simulink model "mdl2"  (Simulink 8.1)
settings: Solver=FixedStepDiscrete  SolverMode=SingleTasking  StartTime=TIME(1)  StopTime=TIME(end)  FixedStep=SIMSTEP  RelTol=1e-3
model workspace (MAT data in the model file):
  autoc_mdd_data01 : struct (value not decoded)
PreLoadFcn:
  | run('C:\Users\yoshi12\Documents\lab_yoshi\matlab\20150408_BenchMarkModel\auto_set.m');
  | load('scr_simdata_all.mat');
  | load('scr_simdata.mat');
undefined symbols (not defined in the file): Parameter144, Parameter25, Parameter29, Parameter33, Parameter35, Parameter38, Parameter41, Parameter43, Parameter45, Parameter48, Parameter51, Parameter52, Parameter53, SIMSTEP
libraries: lib_all x9
settings Model: autoc_cdm_savetype=ModelWorkspace  autoc_cdm_name=autoc_mdd_data01  autoc_current_model=mdl2  autoc_dsminitmode=spec  Creator=905900  LastModifiedBy=yoshi12
settings OptimizationCC: BooleanDataType=off  InlineParams=on  InlineInvariantSignals=on  UseTempVars=on  InitFltsAndDblsToZero=on  OptimizeModelRefInitCode=on  LifeSpan=1
settings DebuggingCC: SignalInfNanChecking=warning  SaveWithParameterizedLinksMsg=none  CheckExecutionContextPreStartOutputMsg=on  CheckExecutionContextRuntimeOutputMsg=on  TimeAdjustmentMsg=warning  SolverPrmCheckMsg=none  InheritedTsInSrcMsg=none  MultiTaskDSMMsg=warning  MultiTaskCondExecSysMsg=none  TasksWithSamePriorityMsg=none  UnconnectedInputMsg=error  UnconnectedOutputMsg=error  UnconnectedLineMsg=error  UniqueDataStoreMsg=error  BusObjectLabelMismatch=error  RootOutportRequireBusObject=error  ModelReferenceIOMsg=warning  ModelReferenceVersionMismatchMessage=warning  ModelReferenceIOMismatchMessage=warning  StrictBusMsg=Warning
settings HardwareCC: ProdIntDivRoundTo=Floor  ProdEndianess=LittleEndian  ProdHWDeviceType=Specified  TargetHWDeviceType=32-bit Generic  ProdEqTarget=off
settings ModelReferenceCC: ModelReferenceNumInstancesAllowed=Single
settings SFSimCC: SimParseCustomCode=off
settings RTWCC: SystemTargetFile=ert.tlc  GenCodeOnly=on  TemplateMakefile=ert_default_tmf  Description=Real-Time Workshop Embedded Coder (no auto configuration)  RTWVerbose=off  ProcessScript=ert_make_rtw_hook
settings CodeAppCC: ForceParamTrailComments=on  IgnoreCustomStorageClasses=off  CustomSymbolStrType=$N$R$M  InternalIdentifier=Classic
settings ERTTargetCC: TargetFcnLib=ansi_tfl_tmw.mat  CodeReplacementLibrary=ANSI_C  MultiwordLength=2048  GenerateSampleERTMain=on  InlinedParameterPlacement=NonHierarchical  ERTCustomFileTemplate=example_file_process.tlc  ConvertIfToSwitch=off  SuppressUnreachableDefaultCases=off

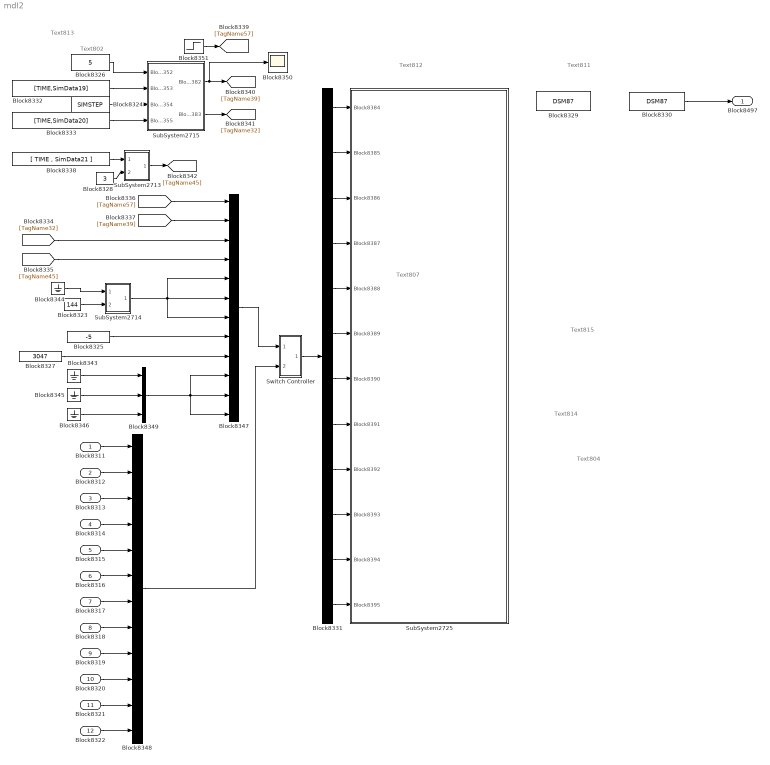
== system mdl2 ==
  note: Text815
  note: Text814
  note: Text813
  note: Text812
  note: Text811
  note: Text807
  note: Text804
  note: Text802
  Block8311 : Inport  SampleTime=SIMSTEP
  Block8312 : Inport  Port=2  SampleTime=SIMSTEP
  Block8313 : Inport  Port=3  PortDimensions=1
  Block8314 : Inport  Port=4  PortDimensions=3
  Block8315 : Inport  Port=5  PortDimensions=144
  Block8316 : Inport  Port=6  PortDimensions=144
  Block8317 : Inport  Port=7  PortDimensions=144
  Block8318 : Inport  Port=8  PortDimensions=1
  Block8319 : Inport  Port=9  PortDimensions=1
  Block8320 : Inport  Port=10  PortDimensions=3
  Block8321 : Inport  Port=11  PortDimensions=3
  Block8322 : Inport  Port=12  PortDimensions=3
  Block8323 : Constant  Value=144  OutDataTypeStr=double  SampleTime=-1
  Block8324 : Constant  Value=SIMSTEP  OutDataTypeStr=double  SampleTime=-1
  Block8325 : Constant  Value=-5  OutDataTypeStr=double  SampleTime=SIMSTEP
  Block8326 : Constant  Value=5  OutDataTypeStr=double  SampleTime=-1
  Block8327 : Constant  Value=3047  OutDataTypeStr=double  SampleTime=-1
  Block8328 : Constant  Value=3  OutDataTypeStr=double  SampleTime=-1
  Block8329 : DataStoreMemory  DataStoreName=DSM87  InitialValue=[0 0 0]  OutDataTypeStr=double
  Block8330 : DataStoreRead  DataStoreName=DSM87
  Block8331 : Demux  Outputs=12
  Block8332 : FromWorkspace  VariableName=[TIME,SimData19]  SampleTime=SIMSTEP
  Block8333 : FromWorkspace  VariableName=[TIME,SimData20]  SampleTime=SIMSTEP  Interpolate=off  OutputAfterFinalValue=Holding final value
  Block8338 : FromWorkspace  VariableName=[ TIME , SimData21 ]  SampleTime=SIMSTEP  Interpolate=off  OutputAfterFinalValue=Holding final value
  Block{8343..8346} (4 alike) : Ground
  Block8347 : Mux  Inputs=12
  Block8348 : Mux  Inputs=12
  Block8349 : Mux  Inputs=3
  Block8350 : Scope
      settings: YMin=0  YMax=1
  Block8351 : Step  Time=SIMSTEP  SampleTime=SIMSTEP
  SubSystem2713 : Subsystem
  SubSystem2714 : Subsystem
  SubSystem2715 : Subsystem
  SubSystem2725 : Subsystem
  Switch Controller : Subsystem  mask(Switch Controller){}
      mask init:
      | if strcmpi(get_param(bdroot(gcbh), 'ModelReferenceTargetType'), 'SIM')
      |     % During simulation, data source for unit model is coming from parent model
      |     mode = false;
      | else
      |     mode = true;
      | end
      | switch_mode = mode;
      settings: OpenFcn="msgbox(['1. モデル単体でのシミュレーション時，In端子を出力します．' 10 10 '2. Model Reference経由で起動時，MR_In端子を出力します．' 10 10 10 '  ■注意：モデルの表紙ページでのみ使用してください．'], 'Switch Controller');"
  Block8497 : Outport
  wires:
  Block8330/1 -> Block8497/1
  Block8331/1 -> SubSystem2725/1(Block8384)
  Block8331/2 -> SubSystem2725/2(Block8385)
  Block8331/3 -> SubSystem2725/3(Block8386)
  Block8331/4 -> SubSystem2725/4(Block8387)
  Block8331/5 -> SubSystem2725/5(Block8388)
  Block8331/6 -> SubSystem2725/6(Block8389)
  Block8331/7 -> SubSystem2725/7(Block8390)
  Block8331/8 -> SubSystem2725/8(Block8391)
  Block8331/9 -> SubSystem2725/9(Block8392)
  Block8331/10 -> SubSystem2725/10(Block8393)
  Block8331/11 -> SubSystem2725/11(Block8394)
  Block8331/12 -> SubSystem2725/12(Block8395)
  Switch Controller/1(Out) -> Block8331/1
  Block8311/1 -> Block8348/1
  Block8312/1 -> Block8348/2
  Block8313/1 -> Block8348/3
  Block8314/1 -> Block8348/4
  Block8315/1 -> Block8348/5
  Block8316/1 -> Block8348/6
  Block8317/1 -> Block8348/7
  Block8318/1 -> Block8348/8
  Block8319/1 -> Block8348/9
  Block8320/1 -> Block8348/10
  Block8321/1 -> Block8348/11
  Block8322/1 -> Block8348/12
  Block8347/1 -> Switch Controller/1(In)
  Block8348/1 -> Switch Controller/2(MR_In)
  [TagName45] -> Block8347/4
  Block8327/1 -> Block8347/9
  [TagName32] -> Block8347/3
  Block8325/1 -> Block8347/8
  Block8343/1 -> Block8349/1
  Block8345/1 -> Block8349/2
  Block8346/1 -> Block8349/3
  Block8349/1 -> Block8347/11, Block8347/10, Block8347/12
  Block8338/1 -> SubSystem2713/1(Scalar)
  SubSystem2713/1(Vector) -> [TagName45]
  Block8328/1 -> SubSystem2713/2(Width)
  [TagName57] -> Block8347/1
  [TagName39] -> Block8347/2
  SubSystem2714/1(Vector) -> Block8347/6, Block8347/7, Block8347/5
  Block8344/1 -> SubSystem2714/1(Scalar)
  Block8323/1 -> SubSystem2714/2(Width)
  Block8351/1 -> [TagName57]
  Block8332/1 -> SubSystem2715/2(Block8353)
  Block8324/1 -> SubSystem2715/3(Block8354)
  SubSystem2715/2(Block8383) -> [TagName32]
  Block8333/1 -> SubSystem2715/4(Block8355)
  Block8326/1 -> SubSystem2715/1(Block8352)
  SubSystem2715/1(Block8382) -> [TagName39], Block8350/1

== system mdl2/SubSystem2713 ==
  note: ***編集禁止***
  Scalar : Inport
  Width : Inport  Port=2
  Mux : Mux  Inputs=3
  Terminator : Terminator
  Vector : Outport
  wires:
  Width/1 -> Terminator/1
  Mux/1 -> Vector/1
  Scalar/1 -> Mux/1, Mux/2, Mux/3

== system mdl2/SubSystem2714 ==
  note: ***編集禁止***
  Scalar : Inport
  Width : Inport  Port=2
  Mux : Mux  Inputs=144
  Terminator : Terminator
  Vector : Outport
  wires:
  Mux/1 -> Vector/1
  Width/1 -> Terminator/1
  Scalar/1 -> Mux/1, Mux/2, Mux/3, Mux/4, Mux/5, Mux/6, Mux/7, Mux/8, Mux/9, Mux/10, Mux/11, Mux/12, Mux/13, Mux/14, Mux/15, Mux/16, Mux/17, Mux/18, Mux/19, Mux/20, Mux/21, Mux/22, Mux/23, Mux/24, Mux/25, Mux/26, Mux/27, Mux/28, Mux/29, Mux/30, Mux/31, Mux/32, Mux/33, Mux/34, Mux/35, Mux/36, Mux/37, Mux/38, Mux/39, Mux/40, Mux/41, Mux/42, Mux/43, Mux/44, Mux/45, Mux/46, Mux/47, Mux/48, Mux/49, Mux/50, Mux/51, Mux/52, Mux/53, Mux/54, Mux/55, Mux/56, Mux/57, Mux/58, Mux/59, Mux/60, Mux/61, Mux/62, Mux/63, Mux/64, Mux/65, Mux/66, Mux/67, Mux/68, Mux/69, Mux/70, Mux/71, Mux/72, Mux/73, Mux/74, Mux/75, Mux/76, Mux/77, Mux/78, Mux/79, Mux/80, Mux/81, Mux/82, Mux/83, Mux/84, Mux/85, Mux/86, Mux/87, Mux/88, Mux/89, Mux/90, Mux/91, Mux/92, Mux/93, Mux/94, Mux/95, Mux/96, Mux/97, Mux/98, Mux/99, Mux/100, Mux/101, Mux/102, Mux/103, Mux/104, Mux/105, Mux/106, Mux/107, Mux/108, Mux/109, Mux/110, Mux/111, Mux/112, Mux/113, Mux/114, Mux/115, Mux/116, Mux/117, Mux/118, Mux/119, Mux/120, Mux/121, Mux/122, Mux/123, Mux/124, Mux/125, Mux/126, Mux/127, Mux/128, Mux/129, Mux/130, Mux/131, Mux/132, Mux/133, Mux/134, Mux/135, Mux/136, Mux/137, Mux/138, Mux/139, Mux/140, Mux/141, Mux/142, Mux/143, Mux/144

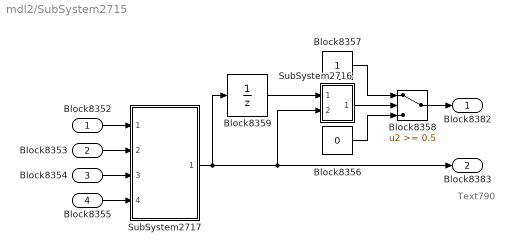
== system mdl2/SubSystem2715 ==
  note: Text790
  Block8352 : Inport
  Block8353 : Inport  Port=2
  Block8354 : Inport  Port=3
  Block8355 : Inport  Port=4
  Block8356 : Constant  Value=0  OutDataTypeStr=double  SampleTime=-1
  Block8357 : Constant  OutDataTypeStr=double  SampleTime=-1
  Block8358 : Switch  Threshold=0.5  RndMeth=Zero  SaturateOnIntegerOverflow=on  InputSameDT=on
  Block8359 : UnitDelay  SampleTime=-1
  SubSystem2716 : Subsystem
  SubSystem2717 : Subsystem
  Block8382 : Outport
  Block8383 : Outport  Port=2
  wires:
  SubSystem2717/1(Block8381) -> Block8359/1, Block8383/1, SubSystem2716/2(In2)
  Block8359/1 -> SubSystem2716/1(In1)
  SubSystem2716/1(Out1) -> Block8358/2
  Block8357/1 -> Block8358/1
  Block8356/1 -> Block8358/3
  Block8358/1 -> Block8382/1
  Block8353/1 -> SubSystem2717/2(Block8361)
  Block8354/1 -> SubSystem2717/3(Block8362)
  Block8355/1 -> SubSystem2717/4(Block8363)
  Block8352/1 -> SubSystem2717/1(Block8360)

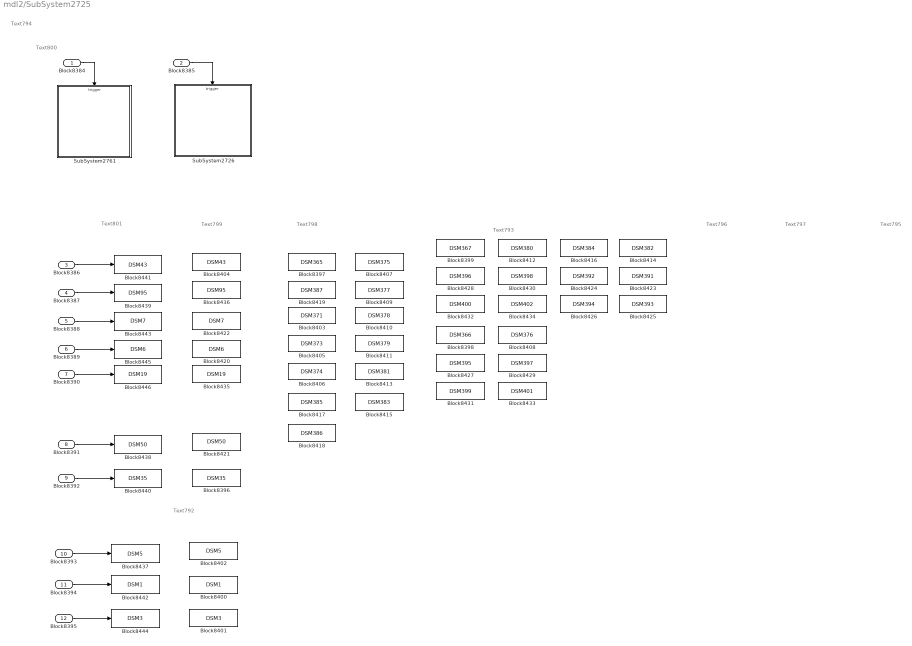
== system mdl2/SubSystem2725 ==
  note: Text801
  note: Text800
  note: Text799
  note: Text798
  note: Text797
  note: Text796
  note: Text795
  note: Text794
  note: Text793
  note: Text792
  Block8384 : Inport
  Block8385 : Inport  Port=2
  Block8386 : Inport  Port=3
  Block8387 : Inport  Port=4
  Block8388 : Inport  Port=5
  Block8389 : Inport  Port=6
  Block8390 : Inport  Port=7
  Block8391 : Inport  Port=8
  Block8392 : Inport  Port=9
  Block8393 : Inport  Port=10
  Block8394 : Inport  Port=11
  Block8395 : Inport  Port=12
  Block8396 : DataStoreMemory  DataStoreName=DSM35  OutDataTypeStr=double
  Block8397 : DataStoreMemory  DataStoreName=DSM365  OutDataTypeStr=double
  Block8398 : DataStoreMemory  DataStoreName=DSM366  InitialValue=[0 0 0 0 0 0 0 0 0 0 0 0 0 0 0 0 0 0 0 0 0 0 0 0 0 0 0 0 0 0 0 0 0 0 0 0 0 0 0 0 0 0 0 0 0 0 0 0 0 0 0 0 0 0 0 0 0 0 0 0 0 0 0 0 0 0 0 0 0 0 0 0 0 0 0 0 0 0 0 0 0 0 0 0 0 0 0 0 0 0 0 0 0 0 0 0 0 0 0 0 0 0 0 0 0 0 0 0 0 0 0 0 0 0 0 0 0 0 0 0 0 0 0 0 0 0 0 0]  OutDataTypeStr=double
  Block8399 : DataStoreMemory  DataStoreName=DSM367  InitialValue=[0 0 0 0 0 0 0 0 0 0 0 0 0 0 0 0 0 0 0 0 0 0 0 0 0 0 0 0 0 0 0 0 0 0 0 0 0 0 0 0 0 0 0 0 0 0 0 0 0 0 0 0 0 0 0 0 0 0 0 0 0 0 0 0 0 0 0 0 0 0 0 0 0 0 0 0 0 0 0 0 0 0 0 0 0 0 0 0 0 0 0 0 0 0 0 0 0 0 0 0 0 0 0 0 0 0 0 0 0 0 0 0 0 0 0 0 0 0 0 0 0 0 0 0 0 0 0 0]  OutDataTypeStr=double
  Block8400 : DataStoreMemory  DataStoreName=DSM1  InitialValue=[0 0 0]  OutDataTypeStr=double
  Block8401 : DataStoreMemory  DataStoreName=DSM3  InitialValue=[0 0 0]  OutDataTypeStr=double
  Block8402 : DataStoreMemory  DataStoreName=DSM5  InitialValue=[0 0 0]  OutDataTypeStr=double
  Block8403 : DataStoreMemory  DataStoreName=DSM371  InitialValue=[0 0 0]  OutDataTypeStr=double
  Block8404 : DataStoreMemory  DataStoreName=DSM43  OutDataTypeStr=double
  Block8405 : DataStoreMemory  DataStoreName=DSM373  InitialValue=[0 0 0]  OutDataTypeStr=double
  Block8406 : DataStoreMemory  DataStoreName=DSM374  InitialValue=[0 0 0]  OutDataTypeStr=double
  Block8407 : DataStoreMemory  DataStoreName=DSM375  InitialValue=[0 0 0]  OutDataTypeStr=double
  Block8408 : DataStoreMemory  DataStoreName=DSM376  InitialValue=[0 0 0 0 0 0 0 0 0 0 0 0 0 0 0 0]  OutDataTypeStr=double
  Block8409 : DataStoreMemory  DataStoreName=DSM377  InitialValue=[0 0 0]  OutDataTypeStr=double
  Block8410 : DataStoreMemory  DataStoreName=DSM378  InitialValue=[0 0 0]  OutDataTypeStr=double
  Block8411 : DataStoreMemory  DataStoreName=DSM379  InitialValue=[0 0 0]  OutDataTypeStr=double
  Block8412 : DataStoreMemory  DataStoreName=DSM380  InitialValue=[0 0 0 0 0 0 0 0 0 0 0 0 0 0 0 0]  OutDataTypeStr=double
  Block8413 : DataStoreMemory  DataStoreName=DSM381  InitialValue=[0 0 0]  OutDataTypeStr=double
  Block8414 : DataStoreMemory  DataStoreName=DSM382  InitialValue=[0 0 0 0 0 0 0 0 0 0 0 0 0 0 0 0 0 0 0 0 0 0 0 0 0 0 0 0 0 0 0 0 0 0 0 0 0 0 0 0 0 0 0 0 0 0 0 0 0 0 0 0 0 0 0 0 0 0 0 0 0 0 0 0 0 0 0 0 0 0 0 0 0 0 0 0 0 0 0 0 0 0 0 0 0 0 0 0 0 0 0 0 0 0 0 0 0 0 0 0 0 0 0 0 0 0 0 0 0 0 0 0 0 0 0 0 0 0 0 0 0 0 0 0 0 0 0 0]  OutDataTypeStr=double
  Block8415 : DataStoreMemory  DataStoreName=DSM383  InitialValue=[0 0 0]  OutDataTypeStr=double
  Block8416 : DataStoreMemory  DataStoreName=DSM384  InitialValue=[0 0 0 0 0 0 0 0 0 0 0 0 0 0 0 0 0 0 0 0 0 0 0 0 0 0 0 0 0 0 0 0 0 0 0 0 0 0 0 0 0 0 0 0 0 0 0 0 0 0 0 0 0 0 0 0 0 0 0 0 0 0 0 0 0 0 0 0 0 0 0 0 0 0 0 0 0 0 0 0 0 0 0 0 0 0 0 0 0 0 0 0 0 0 0 0 0 0 0 0 0 0 0 0 0 0 0 0 0 0 0 0 0 0 0 0 0 0 0 0 0 0 0 0 0 0 0 0]  OutDataTypeStr=double
  Block8417 : DataStoreMemory  DataStoreName=DSM385  InitialValue=[0 0 0]  OutDataTypeStr=double
  Block8418 : DataStoreMemory  DataStoreName=DSM386  InitialValue=[0 0 0]  OutDataTypeStr=double
  Block8419 : DataStoreMemory  DataStoreName=DSM387  InitialValue=[0 0 0]  OutDataTypeStr=double
  Block8420 : DataStoreMemory  DataStoreName=DSM6  InitialValue=[0 0 0 0 0 0 0 0 0 0 0 0 0 0 0 0 0 0 0 0 0 0 0 0 0 0 0 0 0 0 0 0 0 0 0 0 0 0 0 0 0 0 0 0 0 0 0 0 0 0 0 0 0 0 0 0 0 0 0 0 0 0 0 0 0 0 0 0 0 0 0 0 0 0 0 0 0 0 0 0 0 0 0 0 0 0 0 0 0 0 0 0 0 0 0 0 0 0 0 0 0 0 0 0 0 0 0 0 0 0 0 0 0 0 0 0 0 0 0 0 0 0 0 0 0 0 0 0 0 0 0 0 0 0 0 0 0 0 0 0 0 0 0 0]  OutDataTypeStr=double
  Block8421 : DataStoreMemory  DataStoreName=DSM50  OutDataTypeStr=double
  Block8422 : DataStoreMemory  DataStoreName=DSM7  InitialValue=[0 0 0 0 0 0 0 0 0 0 0 0 0 0 0 0 0 0 0 0 0 0 0 0 0 0 0 0 0 0 0 0 0 0 0 0 0 0 0 0 0 0 0 0 0 0 0 0 0 0 0 0 0 0 0 0 0 0 0 0 0 0 0 0 0 0 0 0 0 0 0 0 0 0 0 0 0 0 0 0 0 0 0 0 0 0 0 0 0 0 0 0 0 0 0 0 0 0 0 0 0 0 0 0 0 0 0 0 0 0 0 0 0 0 0 0 0 0 0 0 0 0 0 0 0 0 0 0 0 0 0 0 0 0 0 0 0 0 0 0 0 0 0 0]  OutDataTypeStr=double
  Block8423 : DataStoreMemory  DataStoreName=DSM391  InitialValue=[0 0 0 0 0 0 0 0 0 0 0 0 0 0 0 0 0 0 0 0 0 0 0 0 0 0 0 0 0 0 0 0 0 0 0 0 0 0 0 0 0 0 0 0 0 0 0 0 0 0 0 0 0 0 0 0 0 0 0 0 0 0 0 0 0 0 0 0 0 0 0 0 0 0 0 0 0 0 0 0 0 0 0 0 0 0 0 0 0 0 0 0 0 0 0 0 0 0 0 0 0 0 0 0 0 0 0 0 0 0 0 0 0 0 0 0 0 0 0 0 0 0 0 0 0 0 0 0]  OutDataTypeStr=double
  Block8424 : DataStoreMemory  DataStoreName=DSM392  InitialValue=[0 0 0 0 0 0 0 0 0 0 0 0 0 0 0 0 0 0 0 0 0 0 0 0 0 0 0 0 0 0 0 0 0 0 0 0 0 0 0 0 0 0 0 0 0 0 0 0 0 0 0 0 0 0 0 0 0 0 0 0 0 0 0 0 0 0 0 0 0 0 0 0 0 0 0 0 0 0 0 0 0 0 0 0 0 0 0 0 0 0 0 0 0 0 0 0 0 0 0 0 0 0 0 0 0 0 0 0 0 0 0 0 0 0 0 0 0 0 0 0 0 0 0 0 0 0 0 0]  OutDataTypeStr=double
  Block8425 : DataStoreMemory  DataStoreName=DSM393  InitialValue=[0 0 0 0 0 0 0 0 0 0 0 0 0 0 0 0 0 0 0 0 0 0 0 0 0 0 0 0 0 0 0 0 0 0 0 0 0 0 0 0 0 0 0 0 0 0 0 0 0 0 0 0 0 0 0 0 0 0 0 0 0 0 0 0 0 0 0 0 0 0 0 0 0 0 0 0 0 0 0 0 0 0 0 0 0 0 0 0 0 0 0 0 0 0 0 0 0 0 0 0 0 0 0 0 0 0 0 0 0 0 0 0 0 0 0 0 0 0 0 0 0 0 0 0 0 0 0 0]  OutDataTypeStr=double
  Block8426 : DataStoreMemory  DataStoreName=DSM394  InitialValue=[0 0 0 0 0 0 0 0 0 0 0 0 0 0 0 0 0 0 0 0 0 0 0 0 0 0 0 0 0 0 0 0 0 0 0 0 0 0 0 0 0 0 0 0 0 0 0 0 0 0 0 0 0 0 0 0 0 0 0 0 0 0 0 0 0 0 0 0 0 0 0 0 0 0 0 0 0 0 0 0 0 0 0 0 0 0 0 0 0 0 0 0 0 0 0 0 0 0 0 0 0 0 0 0 0 0 0 0 0 0 0 0 0 0 0 0 0 0 0 0 0 0 0 0 0 0 0 0]  OutDataTypeStr=double
  Block8427 : DataStoreMemory  DataStoreName=DSM395  InitialValue=[0 0 0 0 0 0 0 0 0 0 0 0 0 0 0 0 0 0 0 0 0 0 0 0 0 0 0 0 0 0 0 0 0 0 0 0 0 0 0 0 0 0 0 0 0 0 0 0 0 0 0 0 0 0 0 0 0 0 0 0 0 0 0 0 0 0 0 0 0 0 0 0 0 0 0 0 0 0 0 0 0 0 0 0 0 0 0 0 0 0 0 0 0 0 0 0 0 0 0 0 0 0 0 0 0 0 0 0 0 0 0 0 0 0 0 0 0 0 0 0 0 0 0 0 0 0 0 0]  OutDataTypeStr=double
  Block8428 : DataStoreMemory  DataStoreName=DSM396  InitialValue=[0 0 0 0 0 0 0 0 0 0 0 0 0 0 0 0 0 0 0 0 0 0 0 0 0 0 0 0 0 0 0 0 0 0 0 0 0 0 0 0 0 0 0 0 0 0 0 0 0 0 0 0 0 0 0 0 0 0 0 0 0 0 0 0 0 0 0 0 0 0 0 0 0 0 0 0 0 0 0 0 0 0 0 0 0 0 0 0 0 0 0 0 0 0 0 0 0 0 0 0 0 0 0 0 0 0 0 0 0 0 0 0 0 0 0 0 0 0 0 0 0 0 0 0 0 0 0 0]  OutDataTypeStr=double
  Block8429 : DataStoreMemory  DataStoreName=DSM397  InitialValue=[0 0 0 0 0 0 0 0 0 0 0 0 0 0 0 0]  OutDataTypeStr=double
  Block8430 : DataStoreMemory  DataStoreName=DSM398  InitialValue=[0 0 0 0 0 0 0 0 0 0 0 0 0 0 0 0]  OutDataTypeStr=double
  Block8431 : DataStoreMemory  DataStoreName=DSM399  InitialValue=[0 0 0 0 0 0 0 0 0 0 0 0 0 0 0 0 0 0 0 0 0 0 0 0 0 0 0 0 0 0 0 0 0 0 0 0 0 0 0 0 0 0 0 0 0 0 0 0 0 0 0 0 0 0 0 0 0 0 0 0 0 0 0 0 0 0 0 0 0 0 0 0 0 0 0 0 0 0 0 0 0 0 0 0 0 0 0 0 0 0 0 0 0 0 0 0 0 0 0 0 0 0 0 0 0 0 0 0 0 0 0 0 0 0 0 0 0 0 0 0 0 0 0 0 0 0 0 0]  OutDataTypeStr=double
  Block8432 : DataStoreMemory  DataStoreName=DSM400  InitialValue=[0 0 0 0 0 0 0 0 0 0 0 0 0 0 0 0 0 0 0 0 0 0 0 0 0 0 0 0 0 0 0 0 0 0 0 0 0 0 0 0 0 0 0 0 0 0 0 0 0 0 0 0 0 0 0 0 0 0 0 0 0 0 0 0 0 0 0 0 0 0 0 0 0 0 0 0 0 0 0 0 0 0 0 0 0 0 0 0 0 0 0 0 0 0 0 0 0 0 0 0 0 0 0 0 0 0 0 0 0 0 0 0 0 0 0 0 0 0 0 0 0 0 0 0 0 0 0 0]  OutDataTypeStr=double
  Block8433 : DataStoreMemory  DataStoreName=DSM401  InitialValue=[0 0 0 0 0 0 0 0 0 0 0 0 0 0 0 0]  OutDataTypeStr=double
  Block8434 : DataStoreMemory  DataStoreName=DSM402  InitialValue=[0 0 0 0 0 0 0 0 0 0 0 0 0 0 0 0]  OutDataTypeStr=double
  Block8435 : DataStoreMemory  DataStoreName=DSM19  InitialValue=[0 0 0 0 0 0 0 0 0 0 0 0 0 0 0 0 0 0 0 0 0 0 0 0 0 0 0 0 0 0 0 0 0 0 0 0 0 0 0 0 0 0 0 0 0 0 0 0 0 0 0 0 0 0 0 0 0 0 0 0 0 0 0 0 0 0 0 0 0 0 0 0 0 0 0 0 0 0 0 0 0 0 0 0 0 0 0 0 0 0 0 0 0 0 0 0 0 0 0 0 0 0 0 0 0 0 0 0 0 0 0 0 0 0 0 0 0 0 0 0 0 0 0 0 0 0 0 0 0 0 0 0 0 0 0 0 0 0 0 0 0 0 0 0]  OutDataTypeStr=double
  Block8436 : DataStoreMemory  DataStoreName=DSM95  InitialValue=[0 0 0]  OutDataTypeStr=double
  Block8437 : DataStoreWrite  Priority=1  DataStoreName=DSM5
  Block8438 : DataStoreWrite  Priority=1  DataStoreName=DSM50
  Block8439 : DataStoreWrite  Priority=1  DataStoreName=DSM95
  Block8440 : DataStoreWrite  Priority=1  DataStoreName=DSM35
  Block8441 : DataStoreWrite  Priority=1  DataStoreName=DSM43
  Block8442 : DataStoreWrite  Priority=1  DataStoreName=DSM1
  Block8443 : DataStoreWrite  Priority=1  DataStoreName=DSM7
  Block8444 : DataStoreWrite  Priority=1  DataStoreName=DSM3
  Block8445 : DataStoreWrite  Priority=1  DataStoreName=DSM6
  Block8446 : DataStoreWrite  Priority=1  DataStoreName=DSM19
  SubSystem2726 : Subsystem  Priority=3  TreatAsAtomicUnit=on
      settings: AttributesFormatString=Attribute2234  RTWSystemCode=Nonreusable function  RTWFcnNameOpts=Use subsystem name
  SubSystem2761 : Subsystem  Priority=2  TreatAsAtomicUnit=on
      settings: AttributesFormatString=Attribute2268  RTWSystemCode=Nonreusable function  RTWFcnNameOpts=Use subsystem name
  wires:
  Block8385/1 -> SubSystem2726/Trigger
  Block8384/1 -> SubSystem2761/Trigger
  Block8387/1 -> Block8439/1
  Block8386/1 -> Block8441/1
  Block8391/1 -> Block8438/1
  Block8392/1 -> Block8440/1
  Block8388/1 -> Block8443/1
  Block8390/1 -> Block8446/1
  Block8389/1 -> Block8445/1
  Block8393/1 -> Block8437/1
  Block8394/1 -> Block8442/1
  Block8395/1 -> Block8444/1

== system mdl2/Switch Controller ==
  In : Inport  SampleTime=SIMSTEP
  MR_In : Inport  Port=2  SampleTime=SIMSTEP
  Numerical Unity : SignalConversion  ConversionOutput=Bus copy
  Sw1 : Switch  Threshold=0.5  SaturateOnIntegerOverflow=on  InputSameDT=on
  Switch Control : Constant  Value=switch_mode  OutDataTypeStr=boolean
  Out : Outport
  wires:
  In/1 -> Sw1/1
  Switch Control/1 -> Sw1/2
  Sw1/1 -> Numerical Unity/1
  MR_In/1 -> Sw1/3
  Numerical Unity/1 -> Out/1

== system mdl2/SubSystem2715/SubSystem2716 ==
  note: ***編集禁止***
  In1 : Inport
  In2 : Inport  Port=2
  RO1 : RelationalOperator  Operator=~=  InputSameDT=on
  single1 : DataTypeConversion  OutDataTypeStr=single  SaturateOnIntegerOverflow=on  RndMeth=Zero
  single2 : DataTypeConversion  OutDataTypeStr=single  SaturateOnIntegerOverflow=on  RndMeth=Zero
  Out1 : Outport
  wires:
  RO1/1 -> Out1/1
  In2/1 -> single2/1
  In1/1 -> single1/1
  single1/1 -> RO1/1
  single2/1 -> RO1/2

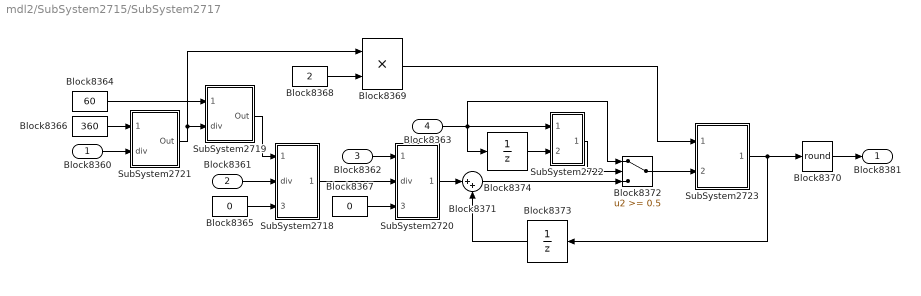
== system mdl2/SubSystem2715/SubSystem2717 ==
  Block8360 : Inport
  Block8361 : Inport  Port=2
  Block8362 : Inport  Port=3
  Block8363 : Inport  Port=4
  Block8364 : Constant  Value=60  OutDataTypeStr=double  SampleTime=-1
  Block8365 : Constant  Value=0  OutDataTypeStr=double  SampleTime=-1
  Block8366 : Constant  Value=360  OutDataTypeStr=double  SampleTime=-1
  Block8367 : Constant  Value=0  OutDataTypeStr=double  SampleTime=-1
  Block8368 : Constant  Value=2  OutDataTypeStr=double  SampleTime=-1
  Block8369 : Product  Inputs=**  SaturateOnIntegerOverflow=on  RndMeth=Zero  InputSameDT=on  OutDataTypeStr=Inherit: Same as first input
  Block8370 : Rounding  Operator=round
  Block8371 : Sum  Inputs=|++  OutDataTypeStr=double  RndMeth=Zero  SaturateOnIntegerOverflow=on  InputSameDT=on
  Block8372 : Switch  Threshold=0.5  RndMeth=Zero  SaturateOnIntegerOverflow=on  InputSameDT=on
  Block8373 : UnitDelay  SampleTime=-1
  Block8374 : UnitDelay  SampleTime=-1
  SubSystem2718 : Subsystem  TreatAsAtomicUnit=on  mask(***ATC.DIVISION***){bd_version=1.01.A, r0=チェック有り, r1=, r2=, r3=, r4=, r5=, r6=, r7=, r8=, r9=, c0=, c1=, c2=, c3=, c4=, c5=, c6=, c7=, c8=, c9=}
      mask prompts: bd_version "Version"
      mask help: これはAutoCからのブロックです．編集禁止．
      settings: OpenFcn=warndlg('変更禁止!');
      mask Help: web(ui_blockhelpmng(gcb));
  SubSystem2719 : Subsystem  TreatAsAtomicUnit=on  mask(***ATC.DIVISION***){bd_version=1.01.A, r0=チェック無し, r1=, r2=, r3=, r4=, r5=, r6=, r7=, r8=, r9=, c0=, c1=, c2=, c3=, c4=, c5=, c6=, c7=, c8=, c9=}
      mask prompts: bd_version "Version"
      mask help: これはAutoCからのブロックです．編集禁止．
      settings: OpenFcn=warndlg('変更禁止!');
      mask Help: web(ui_blockhelpmng(gcb));
  SubSystem2720 : Subsystem  TreatAsAtomicUnit=on  mask(***ATC.DIVISION***){bd_version=1.01.A, r0=チェック有り, r1=, r2=, r3=, r4=, r5=, r6=, r7=, r8=, r9=, c0=, c1=, c2=, c3=, c4=, c5=, c6=, c7=, c8=, c9=}
      mask prompts: bd_version "Version"
      mask help: これはAutoCからのブロックです．編集禁止．
      settings: OpenFcn=warndlg('変更禁止!');
      mask Help: web(ui_blockhelpmng(gcb));
  SubSystem2721 : Subsystem  TreatAsAtomicUnit=on  mask(***ATC.DIVISION***){bd_version=1.01.A, r0=チェック無し, r1=, r2=, r3=, r4=, r5=, r6=, r7=, r8=, r9=, c0=, c1=, c2=, c3=, c4=, c5=, c6=, c7=, c8=, c9=}
      mask prompts: bd_version "Version"
      mask help: これはAutoCからのブロックです．編集禁止．
      settings: OpenFcn=warndlg('変更禁止!');
      mask Help: web(ui_blockhelpmng(gcb));
  SubSystem2722 : Subsystem
  SubSystem2723 : Subsystem
      settings: RTWSystemCode=Inline
  Block8381 : Outport
  wires:
  Block8373/1 -> Block8371/2
  Block8371/1 -> Block8372/3
  Block8361/1 -> SubSystem2718/2(div)
  Block8365/1 -> SubSystem2718/3(init)
  Block8364/1 -> SubSystem2719/1(mult)
  SubSystem2719/1(Out) -> SubSystem2718/1(mult)
  SubSystem2720/1(Out) -> Block8371/1
  Block8362/1 -> SubSystem2720/1(mult)
  SubSystem2718/1(Out) -> SubSystem2720/2(div)
  Block8367/1 -> SubSystem2720/3(init)
  Block8370/1 -> Block8381/1
  SubSystem2722/1(Out1) -> Block8372/2
  Block8363/1 -> SubSystem2722/1(In1), Block8374/1, Block8372/1
  Block8374/1 -> SubSystem2722/2(In2)
  Block8372/1 -> SubSystem2723/2(Block8376)
  SubSystem2723/1(Block8380) -> Block8370/1, Block8373/1
  Block8366/1 -> SubSystem2721/1(mult)
  Block8360/1 -> SubSystem2721/2(div)
  Block8368/1 -> Block8369/2
  SubSystem2721/1(Out) -> SubSystem2719/2(div), Block8369/1
  Block8369/1 -> SubSystem2723/1(Block8375)

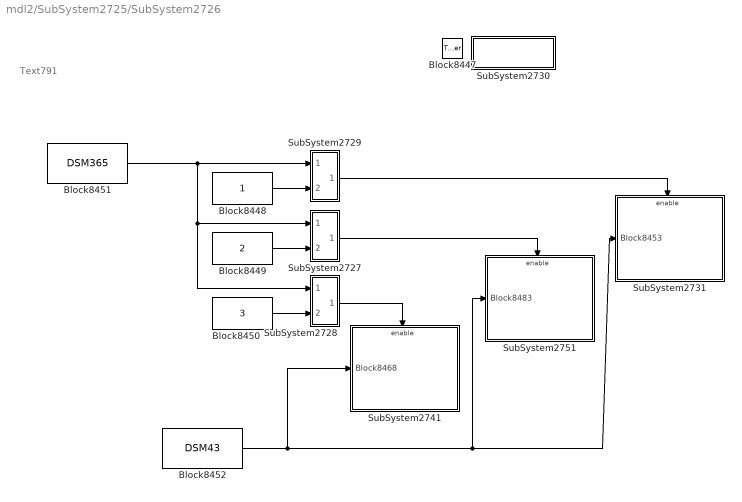
== system mdl2/SubSystem2725/SubSystem2726 ==
  note: Text791
  Block8447 : TriggerPort
  Block8448 : Constant  OutDataTypeStr=double  SampleTime=-1
  Block8449 : Constant  Value=2  OutDataTypeStr=double  SampleTime=-1
  Block8450 : Constant  Value=3  OutDataTypeStr=double  SampleTime=-1
  Block8451 : DataStoreRead  DataStoreName=DSM365
  Block8452 : DataStoreRead  DataStoreName=DSM43
  SubSystem2727 : Subsystem
  SubSystem2728 : Subsystem
  SubSystem2729 : Subsystem
  SubSystem2730 : Subsystem  mask(***ATC.TriggerFunction***){}
      mask help: これはAutoCからのブロックです．編集禁止．
      settings: AttributesFormatString=Attribute2238  OpenFcn=warndlg('変更禁止!');
      mask Display: disp('ATC.Trigger Function')
  SubSystem2731 : Subsystem  TreatAsAtomicUnit=on
  SubSystem2741 : Subsystem  TreatAsAtomicUnit=on
  SubSystem2751 : Subsystem  TreatAsAtomicUnit=on
  wires:
  Block8452/1 -> SubSystem2731/1(Block8453), SubSystem2751/1(Block8483), SubSystem2741/1(Block8468)
  Block8451/1 -> SubSystem2727/1(In1), SubSystem2728/1(In1), SubSystem2729/1(In1)
  Block8448/1 -> SubSystem2729/2(In2)
  Block8449/1 -> SubSystem2727/2(In2)
  Block8450/1 -> SubSystem2728/2(In2)
  SubSystem2729/1(Out1) -> SubSystem2731/Enable
  SubSystem2727/1(Out1) -> SubSystem2751/Enable
  SubSystem2728/1(Out1) -> SubSystem2741/Enable

== system mdl2/SubSystem2725/SubSystem2761 ==
  Block8494 : TriggerPort
  Block8495 : Constant  Value=[1 1 1]  OutDataTypeStr=double  SampleTime=-1
  Block8496 : DataStoreWrite  Priority=1  DataStoreName=DSM87
  SubSystem2762 : Subsystem  mask(***ATC.TriggerFunction***){}
      mask help: これはAutoCからのブロックです．編集禁止．
      settings: AttributesFormatString=Attribute2270  OpenFcn=warndlg('変更禁止!');
      mask Display: disp('ATC.Trigger Function')
  wires:
  Block8495/1 -> Block8496/1

== system mdl2/SubSystem2715/SubSystem2717/SubSystem2718 ==
  note: ***編集禁止***
  mult : Inport
  div : Inport  Port=2
  init : Inport  Port=3
  Product : Subsystem  TreatAsAtomicUnit=on
      settings: RTWSystemCode=Inline
  Out : Outport
  wires:
  Product/1(Out) -> Out/1
  mult/1 -> Product/1(mult)
  div/1 -> Product/2(div)
  init/1 -> Product/3(init)

== system mdl2/SubSystem2715/SubSystem2717/SubSystem2719 ==
  note: ***編集禁止***
  mult : Inport
  div : Inport  Port=2
  Product : Product  Inputs=*/  SaturateOnIntegerOverflow=on  RndMeth=Zero  InputSameDT=on  OutDataTypeStr=Inherit: Same as first input
  Out : Outport
  wires:
  Product/1 -> Out/1
  mult/1 -> Product/1
  div/1 -> Product/2

== system mdl2/SubSystem2715/SubSystem2717/SubSystem2720 ==
  note: ***編集禁止***
  mult : Inport
  div : Inport  Port=2
  init : Inport  Port=3
  Product : Subsystem  TreatAsAtomicUnit=on
      settings: RTWSystemCode=Inline
  Out : Outport
  wires:
  init/1 -> Product/3(init)
  div/1 -> Product/2(div)
  mult/1 -> Product/1(mult)
  Product/1(Out) -> Out/1

== system mdl2/SubSystem2715/SubSystem2717/SubSystem2721 ==
  note: ***編集禁止***
  mult : Inport
  div : Inport  Port=2
  Product : Product  Inputs=*/  SaturateOnIntegerOverflow=on  RndMeth=Zero  InputSameDT=on  OutDataTypeStr=Inherit: Same as first input
  Out : Outport
  wires:
  div/1 -> Product/2
  mult/1 -> Product/1
  Product/1 -> Out/1

== system mdl2/SubSystem2715/SubSystem2717/SubSystem2722 ==
  note: ***編集禁止***
  In1 : Inport
  In2 : Inport  Port=2
  RO1 : RelationalOperator  Operator=~=  InputSameDT=on
  single1 : DataTypeConversion  OutDataTypeStr=single  SaturateOnIntegerOverflow=on  RndMeth=Zero
  single2 : DataTypeConversion  OutDataTypeStr=single  SaturateOnIntegerOverflow=on  RndMeth=Zero
  Out1 : Outport
  wires:
  single2/1 -> RO1/2
  single1/1 -> RO1/1
  In1/1 -> single1/1
  In2/1 -> single2/1
  RO1/1 -> Out1/1

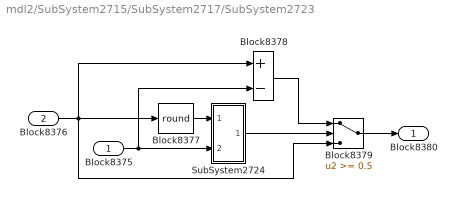
== system mdl2/SubSystem2715/SubSystem2717/SubSystem2723 ==
  Block8375 : Inport
  Block8376 : Inport  Port=2
  Block8377 : Rounding  Operator=round
  Block8378 : Sum  Inputs=+-  OutDataTypeStr=double  RndMeth=Zero  SaturateOnIntegerOverflow=on  InputSameDT=on
  Block8379 : Switch  Threshold=0.5  RndMeth=Zero  SaturateOnIntegerOverflow=on  InputSameDT=on
  SubSystem2724 : Subsystem
  Block8380 : Outport
  wires:
  Block8376/1 -> Block8378/1, Block8379/3, Block8377/1
  Block8375/1 -> Block8378/2, SubSystem2724/2(In2)
  SubSystem2724/1(Out1) -> Block8379/2
  Block8379/1 -> Block8380/1
  Block8378/1 -> Block8379/1
  Block8377/1 -> SubSystem2724/1(In1)

== system mdl2/SubSystem2725/SubSystem2726/SubSystem2727 ==
  note: ***編集禁止***
  In1 : Inport
  In2 : Inport  Port=2
  RO1 : RelationalOperator  Operator===  InputSameDT=on
  single1 : DataTypeConversion  OutDataTypeStr=single  SaturateOnIntegerOverflow=on  RndMeth=Zero
  single2 : DataTypeConversion  OutDataTypeStr=single  SaturateOnIntegerOverflow=on  RndMeth=Zero
  Out1 : Outport
  wires:
  single2/1 -> RO1/2
  single1/1 -> RO1/1
  In1/1 -> single1/1
  In2/1 -> single2/1
  RO1/1 -> Out1/1

== system mdl2/SubSystem2725/SubSystem2726/SubSystem2728 ==
  note: ***編集禁止***
  In1 : Inport
  In2 : Inport  Port=2
  RO1 : RelationalOperator  Operator===  InputSameDT=on
  single1 : DataTypeConversion  OutDataTypeStr=single  SaturateOnIntegerOverflow=on  RndMeth=Zero
  single2 : DataTypeConversion  OutDataTypeStr=single  SaturateOnIntegerOverflow=on  RndMeth=Zero
  Out1 : Outport
  wires:
  single2/1 -> RO1/2
  single1/1 -> RO1/1
  In1/1 -> single1/1
  In2/1 -> single2/1
  RO1/1 -> Out1/1

== system mdl2/SubSystem2725/SubSystem2726/SubSystem2729 ==
  note: ***編集禁止***
  In1 : Inport
  In2 : Inport  Port=2
  RO1 : RelationalOperator  Operator===  InputSameDT=on
  single1 : DataTypeConversion  OutDataTypeStr=single  SaturateOnIntegerOverflow=on  RndMeth=Zero
  single2 : DataTypeConversion  OutDataTypeStr=single  SaturateOnIntegerOverflow=on  RndMeth=Zero
  Out1 : Outport
  wires:
  single2/1 -> RO1/2
  single1/1 -> RO1/1
  In1/1 -> single1/1
  In2/1 -> single2/1
  RO1/1 -> Out1/1

== system mdl2/SubSystem2725/SubSystem2726/SubSystem2730 ==
  note: (Custom TriggerFunction)***編集禁止***<<crank144>>

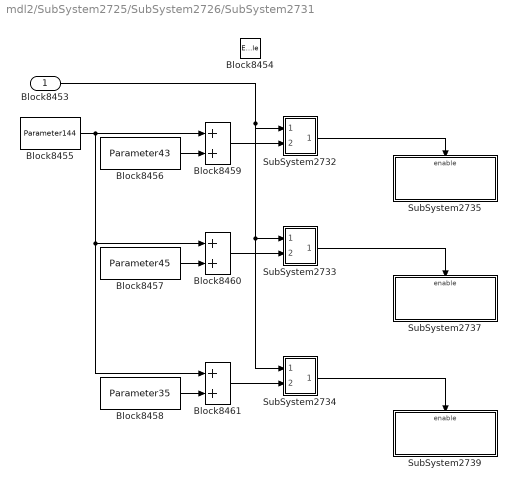
== system mdl2/SubSystem2725/SubSystem2726/SubSystem2731 ==
  Block8453 : Inport
  Block8454 : EnablePort
  Block8455 : Constant  Value=Parameter144  OutDataTypeStr=double  SampleTime=-1
  Block8456 : Constant  Value=Parameter43  OutDataTypeStr=double  SampleTime=-1
  Block8457 : Constant  Value=Parameter45  OutDataTypeStr=double  SampleTime=-1
  Block8458 : Constant  Value=Parameter35  OutDataTypeStr=double  SampleTime=-1
  Block8459 : Sum  OutDataTypeStr=double  RndMeth=Zero  SaturateOnIntegerOverflow=on  InputSameDT=on
  Block8460 : Sum  OutDataTypeStr=double  RndMeth=Zero  SaturateOnIntegerOverflow=on  InputSameDT=on
  Block8461 : Sum  OutDataTypeStr=double  RndMeth=Zero  SaturateOnIntegerOverflow=on  InputSameDT=on
  SubSystem2732 : Subsystem
  SubSystem2733 : Subsystem
  SubSystem2734 : Subsystem
  SubSystem2735 : Subsystem  TreatAsAtomicUnit=on
  SubSystem2737 : Subsystem  TreatAsAtomicUnit=on
  SubSystem2739 : Subsystem  TreatAsAtomicUnit=on
  wires:
  SubSystem2734/1(Out1) -> SubSystem2739/Enable
  SubSystem2733/1(Out1) -> SubSystem2737/Enable
  SubSystem2732/1(Out1) -> SubSystem2735/Enable
  Block8461/1 -> SubSystem2734/2(In2)
  Block8458/1 -> Block8461/2
  Block8460/1 -> SubSystem2733/2(In2)
  Block8457/1 -> Block8460/2
  Block8459/1 -> SubSystem2732/2(In2)
  Block8456/1 -> Block8459/2
  Block8455/1 -> Block8460/1, Block8461/1, Block8459/1
  Block8453/1 -> SubSystem2733/1(In1), SubSystem2734/1(In1), SubSystem2732/1(In1)

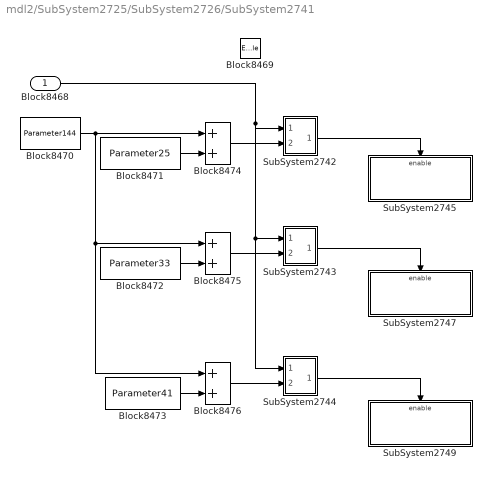
== system mdl2/SubSystem2725/SubSystem2726/SubSystem2741 ==
  Block8468 : Inport
  Block8469 : EnablePort
  Block8470 : Constant  Value=Parameter144  OutDataTypeStr=double  SampleTime=-1
  Block8471 : Constant  Value=Parameter25  OutDataTypeStr=double  SampleTime=-1
  Block8472 : Constant  Value=Parameter33  OutDataTypeStr=double  SampleTime=-1
  Block8473 : Constant  Value=Parameter41  OutDataTypeStr=double  SampleTime=-1
  Block8474 : Sum  OutDataTypeStr=double  RndMeth=Zero  SaturateOnIntegerOverflow=on  InputSameDT=on
  Block8475 : Sum  OutDataTypeStr=double  RndMeth=Zero  SaturateOnIntegerOverflow=on  InputSameDT=on
  Block8476 : Sum  OutDataTypeStr=double  RndMeth=Zero  SaturateOnIntegerOverflow=on  InputSameDT=on
  SubSystem2742 : Subsystem
  SubSystem2743 : Subsystem
  SubSystem2744 : Subsystem
  SubSystem2745 : Subsystem  TreatAsAtomicUnit=on
  SubSystem2747 : Subsystem  TreatAsAtomicUnit=on
  SubSystem2749 : Subsystem  TreatAsAtomicUnit=on
  wires:
  Block8468/1 -> SubSystem2743/1(In1), SubSystem2744/1(In1), SubSystem2742/1(In1)
  Block8470/1 -> Block8474/1, Block8475/1, Block8476/1
  Block8471/1 -> Block8474/2
  Block8474/1 -> SubSystem2742/2(In2)
  Block8472/1 -> Block8475/2
  Block8475/1 -> SubSystem2743/2(In2)
  Block8473/1 -> Block8476/2
  Block8476/1 -> SubSystem2744/2(In2)
  SubSystem2742/1(Out1) -> SubSystem2745/Enable
  SubSystem2743/1(Out1) -> SubSystem2747/Enable
  SubSystem2744/1(Out1) -> SubSystem2749/Enable

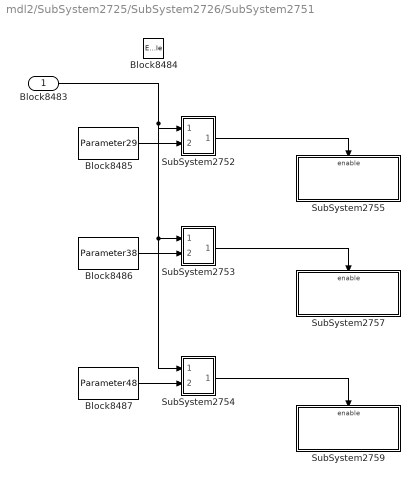
== system mdl2/SubSystem2725/SubSystem2726/SubSystem2751 ==
  Block8483 : Inport
  Block8484 : EnablePort
  Block8485 : Constant  Value=Parameter29  OutDataTypeStr=double  SampleTime=-1
  Block8486 : Constant  Value=Parameter38  OutDataTypeStr=double  SampleTime=-1
  Block8487 : Constant  Value=Parameter48  OutDataTypeStr=double  SampleTime=-1
  SubSystem2752 : Subsystem
  SubSystem2753 : Subsystem
  SubSystem2754 : Subsystem
  SubSystem2755 : Subsystem  TreatAsAtomicUnit=on
  SubSystem2757 : Subsystem  TreatAsAtomicUnit=on
  SubSystem2759 : Subsystem  TreatAsAtomicUnit=on
  wires:
  Block8483/1 -> SubSystem2753/1(In1), SubSystem2754/1(In1), SubSystem2752/1(In1)
  Block8485/1 -> SubSystem2752/2(In2)
  Block8486/1 -> SubSystem2753/2(In2)
  Block8487/1 -> SubSystem2754/2(In2)
  SubSystem2752/1(Out1) -> SubSystem2755/Enable
  SubSystem2753/1(Out1) -> SubSystem2757/Enable
  SubSystem2754/1(Out1) -> SubSystem2759/Enable

== system mdl2/SubSystem2725/SubSystem2761/SubSystem2762 ==
  note: (Custom TriggerFunction)***編集禁止***<<pwon>>

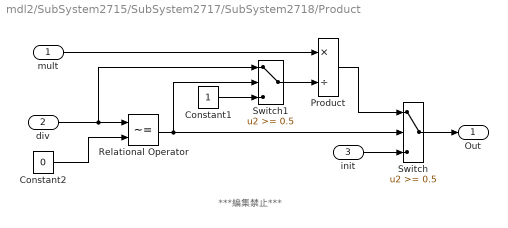
== system mdl2/SubSystem2715/SubSystem2717/SubSystem2718/Product ==
  note: ***編集禁止***
  mult : Inport
  div : Inport  Port=2
  init : Inport  Port=3
  Constant1 : Constant  OutDataTypeStr=Inherit: Inherit via back propagation
  Constant2 : Constant  Value=0  OutDataTypeStr=Inherit: Inherit via back propagation
  Product : Product  Inputs=*/  SaturateOnIntegerOverflow=on  RndMeth=Zero  InputSameDT=on  OutDataTypeStr=Inherit: Same as first input
  Relational Operator : RelationalOperator  Operator=~=  InputSameDT=on
  Switch : Switch  Threshold=0.5  SaturateOnIntegerOverflow=on  InputSameDT=on
  Switch1 : Switch  Threshold=0.5  SaturateOnIntegerOverflow=on  InputSameDT=on
  Out : Outport
  wires:
  Constant1/1 -> Switch1/3
  Constant2/1 -> Relational Operator/2
  Switch1/1 -> Product/2
  div/1 -> Relational Operator/1, Switch1/1
  Switch/1 -> Out/1
  init/1 -> Switch/3
  Relational Operator/1 -> Switch1/2, Switch/2
  Product/1 -> Switch/1
  mult/1 -> Product/1

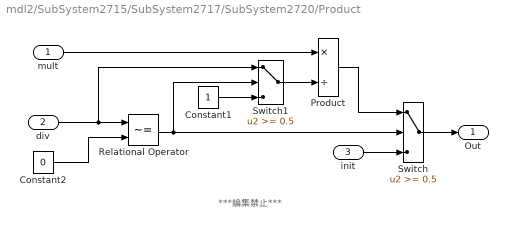
== system mdl2/SubSystem2715/SubSystem2717/SubSystem2720/Product ==
  note: ***編集禁止***
  mult : Inport
  div : Inport  Port=2
  init : Inport  Port=3
  Constant1 : Constant  OutDataTypeStr=Inherit: Inherit via back propagation
  Constant2 : Constant  Value=0  OutDataTypeStr=Inherit: Inherit via back propagation
  Product : Product  Inputs=*/  SaturateOnIntegerOverflow=on  RndMeth=Zero  InputSameDT=on  OutDataTypeStr=Inherit: Same as first input
  Relational Operator : RelationalOperator  Operator=~=  InputSameDT=on
  Switch : Switch  Threshold=0.5  SaturateOnIntegerOverflow=on  InputSameDT=on
  Switch1 : Switch  Threshold=0.5  SaturateOnIntegerOverflow=on  InputSameDT=on
  Out : Outport
  wires:
  Constant1/1 -> Switch1/3
  Constant2/1 -> Relational Operator/2
  Switch1/1 -> Product/2
  div/1 -> Relational Operator/1, Switch1/1
  Switch/1 -> Out/1
  init/1 -> Switch/3
  Relational Operator/1 -> Switch1/2, Switch/2
  Product/1 -> Switch/1
  mult/1 -> Product/1

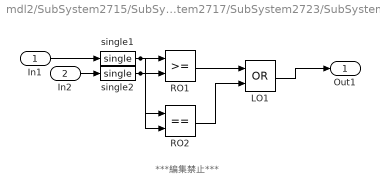
== system mdl2/SubSystem2715/SubSystem2717/SubSystem2723/SubSystem2724 ==
  note: ***編集禁止***
  In1 : Inport
  In2 : Inport  Port=2
  LO1 : Logic  Operator=OR
  RO1 : RelationalOperator  InputSameDT=on
  RO2 : RelationalOperator  Operator===  InputSameDT=on
  single1 : DataTypeConversion  OutDataTypeStr=single  SaturateOnIntegerOverflow=on  RndMeth=Zero
  single2 : DataTypeConversion  OutDataTypeStr=single  SaturateOnIntegerOverflow=on  RndMeth=Zero
  Out1 : Outport
  wires:
  In2/1 -> single2/1
  In1/1 -> single1/1
  single1/1 -> RO1/1, RO2/1
  single2/1 -> RO1/2, RO2/2
  RO1/1 -> LO1/1
  RO2/1 -> LO1/2
  LO1/1 -> Out1/1

== system mdl2/SubSystem2725/SubSystem2726/SubSystem2731/SubSystem2732 ==
  note: ***編集禁止***
  In1 : Inport
  In2 : Inport  Port=2
  RO1 : RelationalOperator  Operator===  InputSameDT=on
  single1 : DataTypeConversion  OutDataTypeStr=single  SaturateOnIntegerOverflow=on  RndMeth=Zero
  single2 : DataTypeConversion  OutDataTypeStr=single  SaturateOnIntegerOverflow=on  RndMeth=Zero
  Out1 : Outport
  wires:
  single2/1 -> RO1/2
  single1/1 -> RO1/1
  In1/1 -> single1/1
  In2/1 -> single2/1
  RO1/1 -> Out1/1

== system mdl2/SubSystem2725/SubSystem2726/SubSystem2731/SubSystem2733 ==
  note: ***編集禁止***
  In1 : Inport
  In2 : Inport  Port=2
  RO1 : RelationalOperator  Operator===  InputSameDT=on
  single1 : DataTypeConversion  OutDataTypeStr=single  SaturateOnIntegerOverflow=on  RndMeth=Zero
  single2 : DataTypeConversion  OutDataTypeStr=single  SaturateOnIntegerOverflow=on  RndMeth=Zero
  Out1 : Outport
  wires:
  single2/1 -> RO1/2
  single1/1 -> RO1/1
  In1/1 -> single1/1
  In2/1 -> single2/1
  RO1/1 -> Out1/1

== system mdl2/SubSystem2725/SubSystem2726/SubSystem2731/SubSystem2734 ==
  note: ***編集禁止***
  In1 : Inport
  In2 : Inport  Port=2
  RO1 : RelationalOperator  Operator===  InputSameDT=on
  single1 : DataTypeConversion  OutDataTypeStr=single  SaturateOnIntegerOverflow=on  RndMeth=Zero
  single2 : DataTypeConversion  OutDataTypeStr=single  SaturateOnIntegerOverflow=on  RndMeth=Zero
  Out1 : Outport
  wires:
  single2/1 -> RO1/2
  single1/1 -> RO1/1
  In1/1 -> single1/1
  In2/1 -> single2/1
  RO1/1 -> Out1/1

== system mdl2/SubSystem2725/SubSystem2726/SubSystem2731/SubSystem2735 ==
  Block8462 : EnablePort
  Block8463 : Constant  Value=Parameter51  OutDataTypeStr=double  SampleTime=-1
  SubSystem2736 : lib_all/SubSystem7  SystemSampleTime=-1
      settings: AttributesFormatString=Attribute2244
  wires:
  Block8463/1 -> SubSystem2736/1

== system mdl2/SubSystem2725/SubSystem2726/SubSystem2731/SubSystem2737 ==
  Block8464 : EnablePort
  Block8465 : Constant  Value=Parameter52  OutDataTypeStr=double  SampleTime=-1
  SubSystem2738 : lib_all/SubSystem7  SystemSampleTime=-1
      settings: AttributesFormatString=Attribute2246
  wires:
  Block8465/1 -> SubSystem2738/1

== system mdl2/SubSystem2725/SubSystem2726/SubSystem2731/SubSystem2739 ==
  Block8466 : EnablePort
  Block8467 : Constant  Value=Parameter53  OutDataTypeStr=double  SampleTime=-1
  SubSystem2740 : lib_all/SubSystem7  SystemSampleTime=-1
      settings: AttributesFormatString=Attribute2248
  wires:
  Block8467/1 -> SubSystem2740/1

== system mdl2/SubSystem2725/SubSystem2726/SubSystem2741/SubSystem2742 ==
  note: ***編集禁止***
  In1 : Inport
  In2 : Inport  Port=2
  RO1 : RelationalOperator  Operator===  InputSameDT=on
  single1 : DataTypeConversion  OutDataTypeStr=single  SaturateOnIntegerOverflow=on  RndMeth=Zero
  single2 : DataTypeConversion  OutDataTypeStr=single  SaturateOnIntegerOverflow=on  RndMeth=Zero
  Out1 : Outport
  wires:
  single2/1 -> RO1/2
  single1/1 -> RO1/1
  In1/1 -> single1/1
  In2/1 -> single2/1
  RO1/1 -> Out1/1

== system mdl2/SubSystem2725/SubSystem2726/SubSystem2741/SubSystem2743 ==
  note: ***編集禁止***
  In1 : Inport
  In2 : Inport  Port=2
  RO1 : RelationalOperator  Operator===  InputSameDT=on
  single1 : DataTypeConversion  OutDataTypeStr=single  SaturateOnIntegerOverflow=on  RndMeth=Zero
  single2 : DataTypeConversion  OutDataTypeStr=single  SaturateOnIntegerOverflow=on  RndMeth=Zero
  Out1 : Outport
  wires:
  single2/1 -> RO1/2
  single1/1 -> RO1/1
  In1/1 -> single1/1
  In2/1 -> single2/1
  RO1/1 -> Out1/1

== system mdl2/SubSystem2725/SubSystem2726/SubSystem2741/SubSystem2744 ==
  note: ***編集禁止***
  In1 : Inport
  In2 : Inport  Port=2
  RO1 : RelationalOperator  Operator===  InputSameDT=on
  single1 : DataTypeConversion  OutDataTypeStr=single  SaturateOnIntegerOverflow=on  RndMeth=Zero
  single2 : DataTypeConversion  OutDataTypeStr=single  SaturateOnIntegerOverflow=on  RndMeth=Zero
  Out1 : Outport
  wires:
  single2/1 -> RO1/2
  single1/1 -> RO1/1
  In1/1 -> single1/1
  In2/1 -> single2/1
  RO1/1 -> Out1/1

== system mdl2/SubSystem2725/SubSystem2726/SubSystem2741/SubSystem2745 ==
  Block8477 : EnablePort
  Block8478 : Constant  Value=Parameter51  OutDataTypeStr=double  SampleTime=-1
  SubSystem2746 : lib_all/SubSystem176  SystemSampleTime=-1
      settings: AttributesFormatString=Attribute2254
  wires:
  Block8478/1 -> SubSystem2746/1

== system mdl2/SubSystem2725/SubSystem2726/SubSystem2741/SubSystem2747 ==
  Block8479 : EnablePort
  Block8480 : Constant  Value=Parameter52  OutDataTypeStr=double  SampleTime=-1
  SubSystem2748 : lib_all/SubSystem176  SystemSampleTime=-1
      settings: AttributesFormatString=Attribute2256
  wires:
  Block8480/1 -> SubSystem2748/1

== system mdl2/SubSystem2725/SubSystem2726/SubSystem2741/SubSystem2749 ==
  Block8481 : EnablePort
  Block8482 : Constant  Value=Parameter53  OutDataTypeStr=double  SampleTime=-1
  SubSystem2750 : lib_all/SubSystem176  SystemSampleTime=-1
      settings: AttributesFormatString=Attribute2258
  wires:
  Block8482/1 -> SubSystem2750/1

== system mdl2/SubSystem2725/SubSystem2726/SubSystem2751/SubSystem2752 ==
  note: ***編集禁止***
  In1 : Inport
  In2 : Inport  Port=2
  RO1 : RelationalOperator  Operator===  InputSameDT=on
  single1 : DataTypeConversion  OutDataTypeStr=single  SaturateOnIntegerOverflow=on  RndMeth=Zero
  single2 : DataTypeConversion  OutDataTypeStr=single  SaturateOnIntegerOverflow=on  RndMeth=Zero
  Out1 : Outport
  wires:
  single2/1 -> RO1/2
  single1/1 -> RO1/1
  In1/1 -> single1/1
  In2/1 -> single2/1
  RO1/1 -> Out1/1

== system mdl2/SubSystem2725/SubSystem2726/SubSystem2751/SubSystem2753 ==
  note: ***編集禁止***
  In1 : Inport
  In2 : Inport  Port=2
  RO1 : RelationalOperator  Operator===  InputSameDT=on
  single1 : DataTypeConversion  OutDataTypeStr=single  SaturateOnIntegerOverflow=on  RndMeth=Zero
  single2 : DataTypeConversion  OutDataTypeStr=single  SaturateOnIntegerOverflow=on  RndMeth=Zero
  Out1 : Outport
  wires:
  single2/1 -> RO1/2
  single1/1 -> RO1/1
  In1/1 -> single1/1
  In2/1 -> single2/1
  RO1/1 -> Out1/1

== system mdl2/SubSystem2725/SubSystem2726/SubSystem2751/SubSystem2754 ==
  note: ***編集禁止***
  In1 : Inport
  In2 : Inport  Port=2
  RO1 : RelationalOperator  Operator===  InputSameDT=on
  single1 : DataTypeConversion  OutDataTypeStr=single  SaturateOnIntegerOverflow=on  RndMeth=Zero
  single2 : DataTypeConversion  OutDataTypeStr=single  SaturateOnIntegerOverflow=on  RndMeth=Zero
  Out1 : Outport
  wires:
  single2/1 -> RO1/2
  single1/1 -> RO1/1
  In1/1 -> single1/1
  In2/1 -> single2/1
  RO1/1 -> Out1/1

== system mdl2/SubSystem2725/SubSystem2726/SubSystem2751/SubSystem2755 ==
  Block8488 : EnablePort
  Block8489 : Constant  Value=Parameter51  OutDataTypeStr=double  SampleTime=-1
  SubSystem2756 : lib_all/SubSystem347  SystemSampleTime=-1
      settings: AttributesFormatString=Attribute2263
  wires:
  Block8489/1 -> SubSystem2756/1

== system mdl2/SubSystem2725/SubSystem2726/SubSystem2751/SubSystem2757 ==
  Block8490 : EnablePort
  Block8491 : Constant  Value=Parameter52  OutDataTypeStr=double  SampleTime=-1
  SubSystem2758 : lib_all/SubSystem347  SystemSampleTime=-1
      settings: AttributesFormatString=Attribute2265
  wires:
  Block8491/1 -> SubSystem2758/1

== system mdl2/SubSystem2725/SubSystem2726/SubSystem2751/SubSystem2759 ==
  Block8492 : EnablePort
  Block8493 : Constant  Value=Parameter53  OutDataTypeStr=double  SampleTime=-1
  SubSystem2760 : lib_all/SubSystem347  SystemSampleTime=-1
      settings: AttributesFormatString=Attribute2267
  wires:
  Block8493/1 -> SubSystem2760/1
